simulink model "proiect_date_modificateV2"  (R2022b)
settings: Solver=VariableStepAuto  StartTime=0.0  StopTime=2500  RelTol=1e-3
values from neighbouring files (symbols this model uses):
  C = 9    [Coeficienti_Pompa.m]    (also in Coeficienti_Pompa_Modificati.m = 5.75; Coeficienti_Pompa_ModificatiV2.m = 7.55)
  k = 0.035    [Coeficienti_Pompa.m]    (also in Coeficienti_Pompa_Modificati.m = 0.025; Coeficienti_Pompa_ModificatiV2.m = 0.037)
  k1 = 0.624    [Coeficienti_Pompa.m]    (also in Coeficienti_Pompa_Modificati.m; Coeficienti_Pompa_ModificatiV2.m)
  k11 = k2^2 + 4* (k - k3) * k1    (= 0.0890826)    [Coeficienti_Pompa.m]    (also in Coeficienti_Pompa_Modificati.m = 0.0641226; Coeficienti_Pompa_ModificatiV2.m = 0.0940746)
  k12 = 8* (k - k3) * h    (= 0.2848)    [Coeficienti_Pompa.m]    (also in Coeficienti_Pompa_Modificati.m = 0.2048; Coeficienti_Pompa_ModificatiV2.m = 0.3008)
  k13 = 2* (k - k3)    (= 0.0712)    [Coeficienti_Pompa.m]    (also in Coeficienti_Pompa_Modificati.m = 0.0512; Coeficienti_Pompa_ModificatiV2.m = 0.0752)
  k2 = -0.015    [Coeficienti_Pompa.m]    (also in Coeficienti_Pompa_Modificati.m; Coeficienti_Pompa_ModificatiV2.m)
  k3 = -0.0006    [Coeficienti_Pompa.m]    (also in Coeficienti_Pompa_Modificati.m; Coeficienti_Pompa_ModificatiV2.m)
  kcompensare = (deltah/deltaq)/(deltah/deltau)    (= 0.1)    [Coeficienti_Pompa.m]    (also in Coeficienti_Pompa_Modificati.m; Coeficienti_Pompa_ModificatiV2.m)
  keta = 8e-5    (= 8e-05)    [Coeficienti_Pompa.m]    (also in Coeficienti_Pompa_Modificati.m; Coeficienti_Pompa_ModificatiV2.m)
libraries: slpidlib x7
(part 1 of 2)
settings Model: Creator=bn19b  LastModifiedBy=bn19b

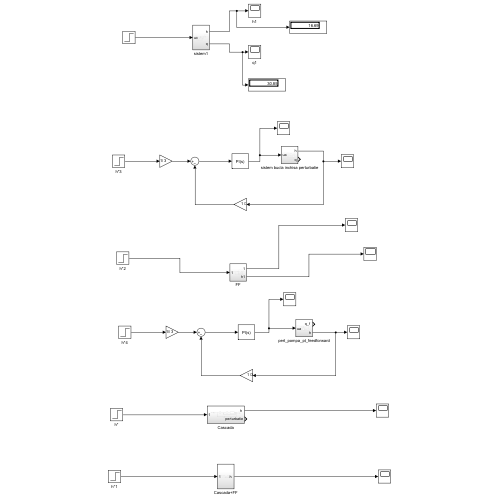
[thumbnail: Simulink's stored preview of the top-level diagram]
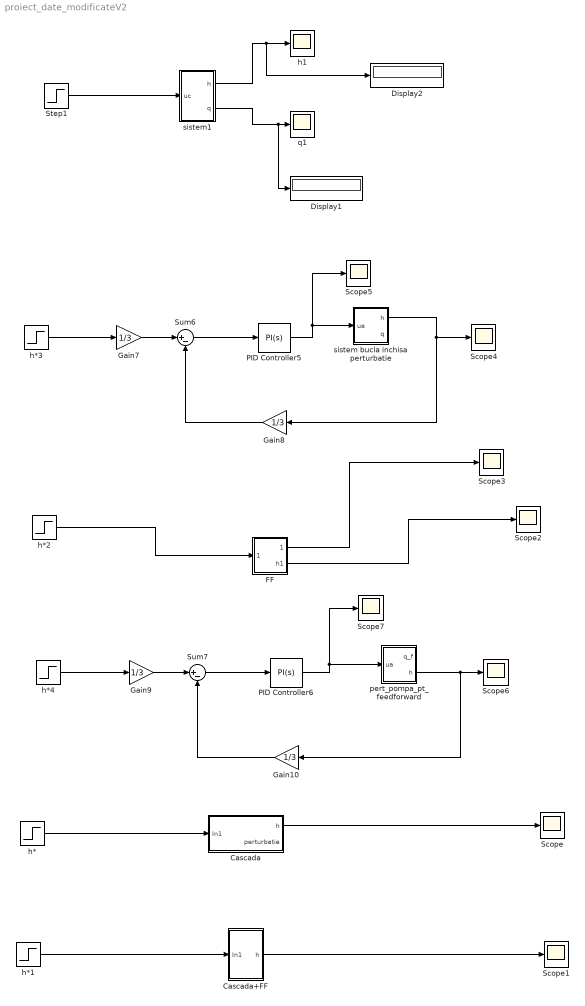
== system proiect_date_modificateV2 ==
  Cascada : Subsystem
  Cascada+FF : Subsystem
  Display1 : Display
  Display2 : Display
  FF : Subsystem
  Gain{7..10} (4 alike) : Gain  Gain=1/3
  PID Controller5 : slpidlib/PID Controller  Controller=PI  Form=Parallel  TimeDomain=Continuous-time  UseExternalTs=off  SampleTime=-1  IntegratorMethod=Forward Euler  FilterMethod=Forward Euler  ControllerParametersSource=internal  P=0.164  I=0.00129  UseKiTs=off  D=0  N=100  UseFilter=on  TunerSelectOption=Transfer Function Based (PID Tuner App)  InitialConditionSource=internal  InitialConditionForIntegrator=5  InitialConditionForFilter=0  DifferentiatorICPrevScaledInput=0  ExternalReset=none  TrackingMode=off  Kt=1  LimitOutput=off  SatLimitsSource=internal  UpperSaturationLimit=inf  LowerSaturationLimit=-inf  LinearizeAsGain=on  AntiWindupMode=none  Kb=1  LimitIntegrator=off  UpperIntegratorSaturationLimit=inf  LowerIntegratorSaturationLimit=-inf  POutMin=[]  POutMax=[]  IOutMin=[]  IOutMax=[]  DOutMin=[]  DOutMax=[]  NOutMin=[]  NOutMax=[]  SumOutMin=[]  SumOutMax=[]  SaturationOutMin=[]  SaturationOutMax=[]  PParamMin=[]  PParamMax=[]  IParamMin=[]  IParamMax=[]  DParamMin=[]  DParamMax=[]  NParamMin=[]  NParamMax=[]  KbParamMin=[]  KbParamMax=[]  KtParamMin=[]  KtParamMax=[]  KbOutMin=[]  KbOutMax=[]  KtOutMin=[]  KtOutMax=[]  IntegratorOutMin=[]  IntegratorOutMax=[]  FilterOutMin=[]  FilterOutMax=[]  SumI1OutMin=[]  SumI1OutMax=[]  SumI2OutMin=[]  SumI2OutMax=[]  SumI3OutMin=[]  SumI3OutMax=[]  SumI4OutMin=[]  SumI4OutMax=[]  SumDOutMin=[]  SumDOutMax=[]  DifferentiatorOutMin=[]  DifferentiatorOutMax=[]  FilterDiffOutCoefMin=[]  FilterDiffOutCoefMax=[]  ReciprocalOutMin=[]  ReciprocalOutMax=[]  SumDenOutMin=[]  SumDenOutMax=[]  SumNumOutMin=[]  SumNumOutMax=[]  DivideOutMin=[]  DivideOutMax=[]  UdiffTsProdOutMin=[]  UdiffTsProdOutMax=[]  NTsProdOutMin=[]  NTsProdOutMax=[]  UintegralTsProdOutMin=[]  UintegralTsProdOutMax=[]  UngainTsProdOutMin=[]  UngainTsProdOutMax=[]  ClampingZeroOutDataTypeStr=Inherit: Inherit via back propagation  ClampingZeroOutMin=[]  ClampingZeroOutMax=[]  FilterDenConstantOutDataTypeStr=Inherit: Inherit via back propagation  FilterDenConstantOutMin=[]  FilterDenConstantOutMax=[]  PCopyOutDataTypeStr=Inherit: Inherit via back propagation  PCopyOutMin=[]  PCopyOutMax=[]  NCopyOutDataTypeStr=Inherit: Inherit via back propagation  NCopyOutMin=[]  NCopyOutMax=[]  IntegratorContinuousStateAttributes=''  IntegratorStateMustResolveToSignalObject=off  IntegratorRTWStateStorageClass=Auto  FilterContinuousStateAttributes=''  FilterStateMustResolveToSignalObject=off  FilterRTWStateStorageClass=Auto  ParallelPVariant=InternalParameters  IdealPVariant=Disabled  IVariant=InternalParameters  DVariant=Disabled  IntegratorVariant=Continuous  SatVariant=Disabled  AWVariant=Passthrough  PCopyVariant=Disabled  TRVariant=Disabled  FdbkBlocksVariant=Forward  IdealPFdbkVariant=Disabled  SatFdbkVariant=Disabled  DerivativeFilterVariant=Disabled  NVariant=Disabled  NCopyVariant=Disabled_SignalSpec  FilterICVariant=Disabled  IntegratorICVariant=InternalICs  ExternalResetVariant=Disabled  TRSumVariant=Passthrough  SumFdbkVariant=Disabled  SumVariant=Sum_PI  TsampFilterVariant=InternalTs  TsampNgainVariant=Passthrough  TsampIntegralVariant=Passthrough  ExternalSaturationOutDataTypeStr=Inherit: Same as second input
  PID Controller6 : slpidlib/PID Controller  Controller=PI  Form=Parallel  TimeDomain=Continuous-time  UseExternalTs=off  SampleTime=-1  IntegratorMethod=Forward Euler  FilterMethod=Forward Euler  ControllerParametersSource=internal  P=0.164  I=0.00129  UseKiTs=off  D=0  N=100  UseFilter=on  TunerSelectOption=Transfer Function Based (PID Tuner App)  InitialConditionSource=internal  InitialConditionForIntegrator=5  InitialConditionForFilter=0  DifferentiatorICPrevScaledInput=0  ExternalReset=none  TrackingMode=off  Kt=1  LimitOutput=off  SatLimitsSource=internal  UpperSaturationLimit=inf  LowerSaturationLimit=-inf  LinearizeAsGain=on  AntiWindupMode=none  Kb=1  LimitIntegrator=off  UpperIntegratorSaturationLimit=inf  LowerIntegratorSaturationLimit=-inf  POutMin=[]  POutMax=[]  IOutMin=[]  IOutMax=[]  DOutMin=[]  DOutMax=[]  NOutMin=[]  NOutMax=[]  SumOutMin=[]  SumOutMax=[]  SaturationOutMin=[]  SaturationOutMax=[]  PParamMin=[]  PParamMax=[]  IParamMin=[]  IParamMax=[]  DParamMin=[]  DParamMax=[]  NParamMin=[]  NParamMax=[]  KbParamMin=[]  KbParamMax=[]  KtParamMin=[]  KtParamMax=[]  KbOutMin=[]  KbOutMax=[]  KtOutMin=[]  KtOutMax=[]  IntegratorOutMin=[]  IntegratorOutMax=[]  FilterOutMin=[]  FilterOutMax=[]  SumI1OutMin=[]  SumI1OutMax=[]  SumI2OutMin=[]  SumI2OutMax=[]  SumI3OutMin=[]  SumI3OutMax=[]  SumI4OutMin=[]  SumI4OutMax=[]  SumDOutMin=[]  SumDOutMax=[]  DifferentiatorOutMin=[]  DifferentiatorOutMax=[]  FilterDiffOutCoefMin=[]  FilterDiffOutCoefMax=[]  ReciprocalOutMin=[]  ReciprocalOutMax=[]  SumDenOutMin=[]  SumDenOutMax=[]  SumNumOutMin=[]  SumNumOutMax=[]  DivideOutMin=[]  DivideOutMax=[]  UdiffTsProdOutMin=[]  UdiffTsProdOutMax=[]  NTsProdOutMin=[]  NTsProdOutMax=[]  UintegralTsProdOutMin=[]  UintegralTsProdOutMax=[]  UngainTsProdOutMin=[]  UngainTsProdOutMax=[]  ClampingZeroOutDataTypeStr=Inherit: Inherit via back propagation  ClampingZeroOutMin=[]  ClampingZeroOutMax=[]  FilterDenConstantOutDataTypeStr=Inherit: Inherit via back propagation  FilterDenConstantOutMin=[]  FilterDenConstantOutMax=[]  PCopyOutDataTypeStr=Inherit: Inherit via back propagation  PCopyOutMin=[]  PCopyOutMax=[]  NCopyOutDataTypeStr=Inherit: Inherit via back propagation  NCopyOutMin=[]  NCopyOutMax=[]  IntegratorContinuousStateAttributes=''  IntegratorStateMustResolveToSignalObject=off  IntegratorRTWStateStorageClass=Auto  FilterContinuousStateAttributes=''  FilterStateMustResolveToSignalObject=off  FilterRTWStateStorageClass=Auto  ParallelPVariant=InternalParameters  IdealPVariant=Disabled  IVariant=InternalParameters  DVariant=Disabled  IntegratorVariant=Continuous  SatVariant=Disabled  AWVariant=Passthrough  PCopyVariant=Disabled  TRVariant=Disabled  FdbkBlocksVariant=Forward  IdealPFdbkVariant=Disabled  SatFdbkVariant=Disabled  DerivativeFilterVariant=Disabled  NVariant=Disabled  NCopyVariant=Disabled_SignalSpec  FilterICVariant=Disabled  IntegratorICVariant=InternalICs  ExternalResetVariant=Disabled  TRSumVariant=Passthrough  SumFdbkVariant=Disabled  SumVariant=Sum_PI  TsampFilterVariant=InternalTs  TsampNgainVariant=Passthrough  TsampIntegralVariant=Passthrough  ExternalSaturationOutDataTypeStr=Inherit: Same as second input
  Scope{,1..7} (8 alike) : Scope
  Step1 : Step  After=5.7  SampleTime=0
  Sum6 : Sum  Inputs=|+-
  Sum7 : Sum  Inputs=|+-
  h*{,1..4} (5 alike) : Step  Before=16.69  After=20.85  SampleTime=0
  h1 : Scope
  pert_pompa_pt_feedforward : Subsystem
  q1 : Scope
  sistem bucla inchisa perturbatie : Subsystem
  sistem1 : Subsystem
  wires:
  Sum6/1 -> PID Controller5/1
  sistem bucla inchisa perturbatie/1(h) -> Gain8/1, Scope4/1
  pert_pompa_pt_feedforward/2(h) -> Gain10/1, Scope6/1
  Gain10/1 -> Sum7/2
  sistem1/2(q) -> Display1/1, q1/1
  PID Controller6/1 -> pert_pompa_pt_feedforward/1(ua), Scope7/1
  h*2/1 -> FF/1(In1)
  PID Controller5/1 -> sistem bucla inchisa perturbatie/1(ua), Scope5/1
  h*3/1 -> Gain7/1
  Sum7/1 -> PID Controller6/1
  Gain7/1 -> Sum6/1
  FF/2(h1) -> Scope2/1
  sistem1/1(h) -> Display2/1, h1/1
  h*4/1 -> Gain9/1
  Gain9/1 -> Sum7/1
  FF/1(Out1) -> Scope3/1
  Step1/1 -> sistem1/1(uc)
  Gain8/1 -> Sum6/2
  h*/1 -> Cascada/1(In1)
  Cascada/1("h ") -> Scope/1
  Cascada+FF/1("h ") -> Scope1/1
  h*1/1 -> Cascada+FF/1(In1)

== system proiect_date_modificateV2/Cascada ==
  In1 : Inport
  Gain : Gain  Gain=1/3
  Gain1 : Gain  Gain=1/3
  PID Controller : slpidlib/PID Controller  Controller=PI  Form=Parallel  TimeDomain=Continuous-time  UseExternalTs=off  SampleTime=-1  IntegratorMethod=Forward Euler  FilterMethod=Forward Euler  ControllerParametersSource=internal  P=0.0189  I=8.46e-05  UseKiTs=off  D=0  N=100  UseFilter=on  TunerSelectOption=Transfer Function Based (PID Tuner App)  InitialConditionSource=internal  InitialConditionForIntegrator=29.2  InitialConditionForFilter=0  DifferentiatorICPrevScaledInput=0  ExternalReset=none  TrackingMode=off  Kt=1  LimitOutput=off  SatLimitsSource=internal  UpperSaturationLimit=inf  LowerSaturationLimit=-inf  LinearizeAsGain=on  AntiWindupMode=none  Kb=1  LimitIntegrator=off  UpperIntegratorSaturationLimit=inf  LowerIntegratorSaturationLimit=-inf  POutMin=[]  POutMax=[]  IOutMin=[]  IOutMax=[]  DOutMin=[]  DOutMax=[]  NOutMin=[]  NOutMax=[]  SumOutMin=[]  SumOutMax=[]  SaturationOutMin=[]  SaturationOutMax=[]  PParamMin=[]  PParamMax=[]  IParamMin=[]  IParamMax=[]  DParamMin=[]  DParamMax=[]  NParamMin=[]  NParamMax=[]  KbParamMin=[]  KbParamMax=[]  KtParamMin=[]  KtParamMax=[]  KbOutMin=[]  KbOutMax=[]  KtOutMin=[]  KtOutMax=[]  IntegratorOutMin=[]  IntegratorOutMax=[]  FilterOutMin=[]  FilterOutMax=[]  SumI1OutMin=[]  SumI1OutMax=[]  SumI2OutMin=[]  SumI2OutMax=[]  SumI3OutMin=[]  SumI3OutMax=[]  SumI4OutMin=[]  SumI4OutMax=[]  SumDOutMin=[]  SumDOutMax=[]  DifferentiatorOutMin=[]  DifferentiatorOutMax=[]  FilterDiffOutCoefMin=[]  FilterDiffOutCoefMax=[]  ReciprocalOutMin=[]  ReciprocalOutMax=[]  SumDenOutMin=[]  SumDenOutMax=[]  SumNumOutMin=[]  SumNumOutMax=[]  DivideOutMin=[]  DivideOutMax=[]  UdiffTsProdOutMin=[]  UdiffTsProdOutMax=[]  NTsProdOutMin=[]  NTsProdOutMax=[]  UintegralTsProdOutMin=[]  UintegralTsProdOutMax=[]  UngainTsProdOutMin=[]  UngainTsProdOutMax=[]  ClampingZeroOutDataTypeStr=Inherit: Inherit via back propagation  ClampingZeroOutMin=[]  ClampingZeroOutMax=[]  FilterDenConstantOutDataTypeStr=Inherit: Inherit via back propagation  FilterDenConstantOutMin=[]  FilterDenConstantOutMax=[]  PCopyOutDataTypeStr=Inherit: Inherit via back propagation  PCopyOutMin=[]  PCopyOutMax=[]  NCopyOutDataTypeStr=Inherit: Inherit via back propagation  NCopyOutMin=[]  NCopyOutMax=[]  IntegratorContinuousStateAttributes=''  IntegratorStateMustResolveToSignalObject=off  IntegratorRTWStateStorageClass=Auto  FilterContinuousStateAttributes=''  FilterStateMustResolveToSignalObject=off  FilterRTWStateStorageClass=Auto  ParallelPVariant=InternalParameters  IdealPVariant=Disabled  IVariant=InternalParameters  DVariant=Disabled  IntegratorVariant=Continuous  SatVariant=Disabled  AWVariant=Passthrough  PCopyVariant=Disabled  TRVariant=Disabled  FdbkBlocksVariant=Forward  IdealPFdbkVariant=Disabled  SatFdbkVariant=Disabled  DerivativeFilterVariant=Disabled  NVariant=Disabled  NCopyVariant=Disabled_SignalSpec  FilterICVariant=Disabled  IntegratorICVariant=InternalICs  ExternalResetVariant=Disabled  TRSumVariant=Passthrough  SumFdbkVariant=Disabled  SumVariant=Sum_PI  TsampFilterVariant=InternalTs  TsampNgainVariant=Passthrough  TsampIntegralVariant=Passthrough  ExternalSaturationOutDataTypeStr=Inherit: Same as second input
  PID Controller2 : slpidlib/PID Controller  Controller=PI  Form=Parallel  TimeDomain=Continuous-time  UseExternalTs=off  SampleTime=-1  IntegratorMethod=Forward Euler  FilterMethod=Forward Euler  ControllerParametersSource=internal  P=4.74  I=6.49  UseKiTs=off  D=0  N=100  UseFilter=on  TunerSelectOption=Transfer Function Based (PID Tuner App)  InitialConditionSource=internal  InitialConditionForIntegrator=uc  InitialConditionForFilter=0  DifferentiatorICPrevScaledInput=0  ExternalReset=none  TrackingMode=off  Kt=1  LimitOutput=off  SatLimitsSource=internal  UpperSaturationLimit=inf  LowerSaturationLimit=-inf  LinearizeAsGain=on  AntiWindupMode=none  Kb=1  LimitIntegrator=off  UpperIntegratorSaturationLimit=inf  LowerIntegratorSaturationLimit=-inf  POutMin=[]  POutMax=[]  IOutMin=[]  IOutMax=[]  DOutMin=[]  DOutMax=[]  NOutMin=[]  NOutMax=[]  SumOutMin=[]  SumOutMax=[]  SaturationOutMin=[]  SaturationOutMax=[]  PParamMin=[]  PParamMax=[]  IParamMin=[]  IParamMax=[]  DParamMin=[]  DParamMax=[]  NParamMin=[]  NParamMax=[]  KbParamMin=[]  KbParamMax=[]  KtParamMin=[]  KtParamMax=[]  KbOutMin=[]  KbOutMax=[]  KtOutMin=[]  KtOutMax=[]  IntegratorOutMin=[]  IntegratorOutMax=[]  FilterOutMin=[]  FilterOutMax=[]  SumI1OutMin=[]  SumI1OutMax=[]  SumI2OutMin=[]  SumI2OutMax=[]  SumI3OutMin=[]  SumI3OutMax=[]  SumI4OutMin=[]  SumI4OutMax=[]  SumDOutMin=[]  SumDOutMax=[]  DifferentiatorOutMin=[]  DifferentiatorOutMax=[]  FilterDiffOutCoefMin=[]  FilterDiffOutCoefMax=[]  ReciprocalOutMin=[]  ReciprocalOutMax=[]  SumDenOutMin=[]  SumDenOutMax=[]  SumNumOutMin=[]  SumNumOutMax=[]  DivideOutMin=[]  DivideOutMax=[]  UdiffTsProdOutMin=[]  UdiffTsProdOutMax=[]  NTsProdOutMin=[]  NTsProdOutMax=[]  UintegralTsProdOutMin=[]  UintegralTsProdOutMax=[]  UngainTsProdOutMin=[]  UngainTsProdOutMax=[]  ClampingZeroOutDataTypeStr=Inherit: Inherit via back propagation  ClampingZeroOutMin=[]  ClampingZeroOutMax=[]  FilterDenConstantOutDataTypeStr=Inherit: Inherit via back propagation  FilterDenConstantOutMin=[]  FilterDenConstantOutMax=[]  PCopyOutDataTypeStr=Inherit: Inherit via back propagation  PCopyOutMin=[]  PCopyOutMax=[]  NCopyOutDataTypeStr=Inherit: Inherit via back propagation  NCopyOutMin=[]  NCopyOutMax=[]  IntegratorContinuousStateAttributes=''  IntegratorStateMustResolveToSignalObject=off  IntegratorRTWStateStorageClass=Auto  FilterContinuousStateAttributes=''  FilterStateMustResolveToSignalObject=off  FilterRTWStateStorageClass=Auto  ParallelPVariant=InternalParameters  IdealPVariant=Disabled  IVariant=InternalParameters  DVariant=Disabled  IntegratorVariant=Continuous  SatVariant=Disabled  AWVariant=Passthrough  PCopyVariant=Disabled  TRVariant=Disabled  FdbkBlocksVariant=Forward  IdealPFdbkVariant=Disabled  SatFdbkVariant=Disabled  DerivativeFilterVariant=Disabled  NVariant=Disabled  NCopyVariant=Disabled_SignalSpec  FilterICVariant=Disabled  IntegratorICVariant=InternalICs  ExternalResetVariant=Disabled  TRSumVariant=Passthrough  SumFdbkVariant=Disabled  SumVariant=Sum_PI  TsampFilterVariant=InternalTs  TsampNgainVariant=Passthrough  TsampIntegralVariant=Passthrough  ExternalSaturationOutDataTypeStr=Inherit: Same as second input
  Sum : Sum  Inputs=|+-
  Sum1 : Sum  Inputs=|+-
  sistem_cascada : Subsystem
  "h " : Outport
  perturbatie : Outport  Port=2
  wires:
  Gain/1 -> Sum/1
  PID Controller/1 -> Sum1/1
  Sum1/1 -> PID Controller2/1
  sistem_cascada/3(q1) -> Sum1/2
  Sum/1 -> PID Controller/1
  sistem_cascada/1("h ") -> "h "/1, Gain1/1
  PID Controller2/1 -> sistem_cascada/1(uc)
  Gain1/1 -> Sum/2
  In1/1 -> Gain/1
  sistem_cascada/2(perturbatie) -> perturbatie/1

== system proiect_date_modificateV2/Cascada+FF ==
  In1 : Inport
  Gain2 : Gain  Gain=1/3
  Gain3 : Gain  Gain=1/3
  PID Controller1 : slpidlib/PID Controller  Controller=PI  Form=Parallel  TimeDomain=Continuous-time  UseExternalTs=off  SampleTime=-1  IntegratorMethod=Forward Euler  FilterMethod=Forward Euler  ControllerParametersSource=internal  P=0.0189  I=8.46e-05  UseKiTs=off  D=0  N=100  UseFilter=on  TunerSelectOption=Transfer Function Based (PID Tuner App)  InitialConditionSource=internal  InitialConditionForIntegrator=29.2  InitialConditionForFilter=0  DifferentiatorICPrevScaledInput=0  ExternalReset=none  TrackingMode=off  Kt=1  LimitOutput=off  SatLimitsSource=internal  UpperSaturationLimit=inf  LowerSaturationLimit=-inf  LinearizeAsGain=on  AntiWindupMode=none  Kb=1  LimitIntegrator=off  UpperIntegratorSaturationLimit=inf  LowerIntegratorSaturationLimit=-inf  POutMin=[]  POutMax=[]  IOutMin=[]  IOutMax=[]  DOutMin=[]  DOutMax=[]  NOutMin=[]  NOutMax=[]  SumOutMin=[]  SumOutMax=[]  SaturationOutMin=[]  SaturationOutMax=[]  PParamMin=[]  PParamMax=[]  IParamMin=[]  IParamMax=[]  DParamMin=[]  DParamMax=[]  NParamMin=[]  NParamMax=[]  KbParamMin=[]  KbParamMax=[]  KtParamMin=[]  KtParamMax=[]  KbOutMin=[]  KbOutMax=[]  KtOutMin=[]  KtOutMax=[]  IntegratorOutMin=[]  IntegratorOutMax=[]  FilterOutMin=[]  FilterOutMax=[]  SumI1OutMin=[]  SumI1OutMax=[]  SumI2OutMin=[]  SumI2OutMax=[]  SumI3OutMin=[]  SumI3OutMax=[]  SumI4OutMin=[]  SumI4OutMax=[]  SumDOutMin=[]  SumDOutMax=[]  DifferentiatorOutMin=[]  DifferentiatorOutMax=[]  FilterDiffOutCoefMin=[]  FilterDiffOutCoefMax=[]  ReciprocalOutMin=[]  ReciprocalOutMax=[]  SumDenOutMin=[]  SumDenOutMax=[]  SumNumOutMin=[]  SumNumOutMax=[]  DivideOutMin=[]  DivideOutMax=[]  UdiffTsProdOutMin=[]  UdiffTsProdOutMax=[]  NTsProdOutMin=[]  NTsProdOutMax=[]  UintegralTsProdOutMin=[]  UintegralTsProdOutMax=[]  UngainTsProdOutMin=[]  UngainTsProdOutMax=[]  ClampingZeroOutDataTypeStr=Inherit: Inherit via back propagation  ClampingZeroOutMin=[]  ClampingZeroOutMax=[]  FilterDenConstantOutDataTypeStr=Inherit: Inherit via back propagation  FilterDenConstantOutMin=[]  FilterDenConstantOutMax=[]  PCopyOutDataTypeStr=Inherit: Inherit via back propagation  PCopyOutMin=[]  PCopyOutMax=[]  NCopyOutDataTypeStr=Inherit: Inherit via back propagation  NCopyOutMin=[]  NCopyOutMax=[]  IntegratorContinuousStateAttributes=''  IntegratorStateMustResolveToSignalObject=off  IntegratorRTWStateStorageClass=Auto  FilterContinuousStateAttributes=''  FilterStateMustResolveToSignalObject=off  FilterRTWStateStorageClass=Auto  ParallelPVariant=InternalParameters  IdealPVariant=Disabled  IVariant=InternalParameters  DVariant=Disabled  IntegratorVariant=Continuous  SatVariant=Disabled  AWVariant=Passthrough  PCopyVariant=Disabled  TRVariant=Disabled  FdbkBlocksVariant=Forward  IdealPFdbkVariant=Disabled  SatFdbkVariant=Disabled  DerivativeFilterVariant=Disabled  NVariant=Disabled  NCopyVariant=Disabled_SignalSpec  FilterICVariant=Disabled  IntegratorICVariant=InternalICs  ExternalResetVariant=Disabled  TRSumVariant=Passthrough  SumFdbkVariant=Disabled  SumVariant=Sum_PI  TsampFilterVariant=InternalTs  TsampNgainVariant=Passthrough  TsampIntegralVariant=Passthrough  ExternalSaturationOutDataTypeStr=Inherit: Same as second input
  PID Controller3 : slpidlib/PID Controller  Controller=PI  Form=Parallel  TimeDomain=Continuous-time  UseExternalTs=off  SampleTime=-1  IntegratorMethod=Forward Euler  FilterMethod=Forward Euler  ControllerParametersSource=internal  P=4.74  I=6.49  UseKiTs=off  D=0  N=100  UseFilter=on  TunerSelectOption=Transfer Function Based (PID Tuner App)  InitialConditionSource=internal  InitialConditionForIntegrator=5  InitialConditionForFilter=0  DifferentiatorICPrevScaledInput=0  ExternalReset=none  TrackingMode=off  Kt=1  LimitOutput=off  SatLimitsSource=internal  UpperSaturationLimit=inf  LowerSaturationLimit=-inf  LinearizeAsGain=on  AntiWindupMode=none  Kb=1  LimitIntegrator=off  UpperIntegratorSaturationLimit=inf  LowerIntegratorSaturationLimit=-inf  POutMin=[]  POutMax=[]  IOutMin=[]  IOutMax=[]  DOutMin=[]  DOutMax=[]  NOutMin=[]  NOutMax=[]  SumOutMin=[]  SumOutMax=[]  SaturationOutMin=[]  SaturationOutMax=[]  PParamMin=[]  PParamMax=[]  IParamMin=[]  IParamMax=[]  DParamMin=[]  DParamMax=[]  NParamMin=[]  NParamMax=[]  KbParamMin=[]  KbParamMax=[]  KtParamMin=[]  KtParamMax=[]  KbOutMin=[]  KbOutMax=[]  KtOutMin=[]  KtOutMax=[]  IntegratorOutMin=[]  IntegratorOutMax=[]  FilterOutMin=[]  FilterOutMax=[]  SumI1OutMin=[]  SumI1OutMax=[]  SumI2OutMin=[]  SumI2OutMax=[]  SumI3OutMin=[]  SumI3OutMax=[]  SumI4OutMin=[]  SumI4OutMax=[]  SumDOutMin=[]  SumDOutMax=[]  DifferentiatorOutMin=[]  DifferentiatorOutMax=[]  FilterDiffOutCoefMin=[]  FilterDiffOutCoefMax=[]  ReciprocalOutMin=[]  ReciprocalOutMax=[]  SumDenOutMin=[]  SumDenOutMax=[]  SumNumOutMin=[]  SumNumOutMax=[]  DivideOutMin=[]  DivideOutMax=[]  UdiffTsProdOutMin=[]  UdiffTsProdOutMax=[]  NTsProdOutMin=[]  NTsProdOutMax=[]  UintegralTsProdOutMin=[]  UintegralTsProdOutMax=[]  UngainTsProdOutMin=[]  UngainTsProdOutMax=[]  ClampingZeroOutDataTypeStr=Inherit: Inherit via back propagation  ClampingZeroOutMin=[]  ClampingZeroOutMax=[]  FilterDenConstantOutDataTypeStr=Inherit: Inherit via back propagation  FilterDenConstantOutMin=[]  FilterDenConstantOutMax=[]  PCopyOutDataTypeStr=Inherit: Inherit via back propagation  PCopyOutMin=[]  PCopyOutMax=[]  NCopyOutDataTypeStr=Inherit: Inherit via back propagation  NCopyOutMin=[]  NCopyOutMax=[]  IntegratorContinuousStateAttributes=''  IntegratorStateMustResolveToSignalObject=off  IntegratorRTWStateStorageClass=Auto  FilterContinuousStateAttributes=''  FilterStateMustResolveToSignalObject=off  FilterRTWStateStorageClass=Auto  ParallelPVariant=InternalParameters  IdealPVariant=Disabled  IVariant=InternalParameters  DVariant=Disabled  IntegratorVariant=Continuous  SatVariant=Disabled  AWVariant=Passthrough  PCopyVariant=Disabled  TRVariant=Disabled  FdbkBlocksVariant=Forward  IdealPFdbkVariant=Disabled  SatFdbkVariant=Disabled  DerivativeFilterVariant=Disabled  NVariant=Disabled  NCopyVariant=Disabled_SignalSpec  FilterICVariant=Disabled  IntegratorICVariant=InternalICs  ExternalResetVariant=Disabled  TRSumVariant=Passthrough  SumFdbkVariant=Disabled  SumVariant=Sum_PI  TsampFilterVariant=InternalTs  TsampNgainVariant=Passthrough  TsampIntegralVariant=Passthrough  ExternalSaturationOutDataTypeStr=Inherit: Same as second input
  Sum2 : Sum  Inputs=|+-
  Sum3 : Sum  Inputs=|++-
  cascada+ff : Subsystem
  "h " : Outport
  wires:
  cascada+ff/2(perturbatie) -> Sum3/2
  Gain3/1 -> Sum2/2
  cascada+ff/1("h ") -> "h "/1, Gain3/1
  Sum3/1 -> PID Controller3/1
  Gain2/1 -> Sum2/1
  cascada+ff/3(q1) -> Sum3/3
  PID Controller3/1 -> cascada+ff/1(uc)
  PID Controller1/1 -> Sum3/1
  Sum2/1 -> PID Controller1/1
  In1/1 -> Gain2/1

== system proiect_date_modificateV2/FF ==
  In1 : Inport
  Gain4 : Gain  Gain=1/3
  Gain5 : Gain  Gain=1/3
  Gain6 : Gain  Gain=kcompensare
  PID Controller4 : slpidlib/PID Controller  Controller=PI  Form=Parallel  TimeDomain=Continuous-time  UseExternalTs=off  SampleTime=-1  IntegratorMethod=Forward Euler  FilterMethod=Forward Euler  ControllerParametersSource=internal  P=0.164  I=0.00129  UseKiTs=off  D=0  N=100  UseFilter=on  TunerSelectOption=Transfer Function Based (PID Tuner App)  InitialConditionSource=internal  InitialConditionForIntegrator=5  InitialConditionForFilter=0  DifferentiatorICPrevScaledInput=0  ExternalReset=none  TrackingMode=off  Kt=1  LimitOutput=off  SatLimitsSource=internal  UpperSaturationLimit=inf  LowerSaturationLimit=-inf  LinearizeAsGain=on  AntiWindupMode=none  Kb=1  LimitIntegrator=off  UpperIntegratorSaturationLimit=inf  LowerIntegratorSaturationLimit=-inf  POutMin=[]  POutMax=[]  IOutMin=[]  IOutMax=[]  DOutMin=[]  DOutMax=[]  NOutMin=[]  NOutMax=[]  SumOutMin=[]  SumOutMax=[]  SaturationOutMin=[]  SaturationOutMax=[]  PParamMin=[]  PParamMax=[]  IParamMin=[]  IParamMax=[]  DParamMin=[]  DParamMax=[]  NParamMin=[]  NParamMax=[]  KbParamMin=[]  KbParamMax=[]  KtParamMin=[]  KtParamMax=[]  KbOutMin=[]  KbOutMax=[]  KtOutMin=[]  KtOutMax=[]  IntegratorOutMin=[]  IntegratorOutMax=[]  FilterOutMin=[]  FilterOutMax=[]  SumI1OutMin=[]  SumI1OutMax=[]  SumI2OutMin=[]  SumI2OutMax=[]  SumI3OutMin=[]  SumI3OutMax=[]  SumI4OutMin=[]  SumI4OutMax=[]  SumDOutMin=[]  SumDOutMax=[]  DifferentiatorOutMin=[]  DifferentiatorOutMax=[]  FilterDiffOutCoefMin=[]  FilterDiffOutCoefMax=[]  ReciprocalOutMin=[]  ReciprocalOutMax=[]  SumDenOutMin=[]  SumDenOutMax=[]  SumNumOutMin=[]  SumNumOutMax=[]  DivideOutMin=[]  DivideOutMax=[]  UdiffTsProdOutMin=[]  UdiffTsProdOutMax=[]  NTsProdOutMin=[]  NTsProdOutMax=[]  UintegralTsProdOutMin=[]  UintegralTsProdOutMax=[]  UngainTsProdOutMin=[]  UngainTsProdOutMax=[]  ClampingZeroOutDataTypeStr=Inherit: Inherit via back propagation  ClampingZeroOutMin=[]  ClampingZeroOutMax=[]  FilterDenConstantOutDataTypeStr=Inherit: Inherit via back propagation  FilterDenConstantOutMin=[]  FilterDenConstantOutMax=[]  PCopyOutDataTypeStr=Inherit: Inherit via back propagation  PCopyOutMin=[]  PCopyOutMax=[]  NCopyOutDataTypeStr=Inherit: Inherit via back propagation  NCopyOutMin=[]  NCopyOutMax=[]  IntegratorContinuousStateAttributes=''  IntegratorStateMustResolveToSignalObject=off  IntegratorRTWStateStorageClass=Auto  FilterContinuousStateAttributes=''  FilterStateMustResolveToSignalObject=off  FilterRTWStateStorageClass=Auto  ParallelPVariant=InternalParameters  IdealPVariant=Disabled  IVariant=InternalParameters  DVariant=Disabled  IntegratorVariant=Continuous  SatVariant=Disabled  AWVariant=Passthrough  PCopyVariant=Disabled  TRVariant=Disabled  FdbkBlocksVariant=Forward  IdealPFdbkVariant=Disabled  SatFdbkVariant=Disabled  DerivativeFilterVariant=Disabled  NVariant=Disabled  NCopyVariant=Disabled_SignalSpec  FilterICVariant=Disabled  IntegratorICVariant=InternalICs  ExternalResetVariant=Disabled  TRSumVariant=Passthrough  SumFdbkVariant=Disabled  SumVariant=Sum_PI  TsampFilterVariant=InternalTs  TsampNgainVariant=Passthrough  TsampIntegralVariant=Passthrough  ExternalSaturationOutDataTypeStr=Inherit: Same as second input
  Sum4 : Sum  Inputs=|+-
  Sum5 : Sum  Inputs=|++
  sistem_feedforward : Subsystem
  Out1 : Outport
  h1 : Outport  Port=2
  wires:
  sistem_feedforward/1(h1) -> h1/1, Gain5/1
  Sum4/1 -> PID Controller4/1
  Gain6/1 -> Sum5/2
  sistem_feedforward/2(perturabtie) -> Gain6/1
  Gain5/1 -> Sum4/2
  Sum5/1 -> Out1/1, sistem_feedforward/1(ua)
  PID Controller4/1 -> Sum5/1
  Gain4/1 -> Sum4/1
  In1/1 -> Gain4/1

== system proiect_date_modificateV2/pert_pompa_pt_feedforward ==
  ua : Inport
  Amplificator : Subsystem
  Curent : Subsystem
  "Filtru " : Subsystem
  Motor : Subsystem
  Randament : Subsystem
  Rezervor : Subsystem
  Step : Step  Time=250  After=0.04  SampleTime=0
  pompa_perturbatie1 : Subsystem
  "q_f " : Outport
  h : Outport  Port=2
  wires:
  Motor/1(kn) -> pompa_perturbatie1/1(kn1)
  pompa_perturbatie1/1(q1) -> "Filtru "/1(q)
  Step/1 -> pompa_perturbatie1/3(perturbatie k)
  Rezervor/1(h) -> h/1, pompa_perturbatie1/2(h1), Curent/1(h)
  "Filtru "/1("q_f ") -> "q_f "/1, Rezervor/1("q "), Randament/1(q), Curent/2(q)
  Curent/1(im) -> Motor/2(im)
  Amplificator/1(um) -> Curent/4(um), Randament/2(um), Motor/1(um)
  Randament/1(eta) -> Curent/3(eta)
  ua/1 -> Amplificator/1(ua)

== system proiect_date_modificateV2/sistem bucla inchisa perturbatie ==
  ua : Inport
  Amplificator : Subsystem
  Curent : Subsystem
  "Filtru " : Subsystem
  Motor : Subsystem
  "Pompa " : Subsystem
  Randament : Subsystem
  Rezervor cu perturbatie : Subsystem
  h : Outport
  q : Outport  Port=2
  wires:
  "Pompa "/1(q) -> "Filtru "/1(q)
  ua/1 -> Amplificator/1(ua)
  Rezervor cu perturbatie/1(h1) -> h/1, "Pompa "/2(h), Curent/1(h)
  Motor/1(kn) -> "Pompa "/1(kn)
  "Filtru "/1("q_f ") -> q/1, Rezervor cu perturbatie/1(q1), Randament/1(q), Curent/2(q)
  Amplificator/1(um) -> Curent/4(um), Randament/2(um), Motor/1(um)
  Curent/1(im) -> Motor/2(im)
  Randament/1(eta) -> Curent/3(eta)

== system proiect_date_modificateV2/sistem1 ==
  uc : Inport
  Amplificator : Subsystem
  Bazin : Subsystem
  Curent rotoric : Subsystem
  Filtru : Subsystem
  Motor : Subsystem
  Pompa : Subsystem
  Randament pompa : Subsystem
  h : Outport
  q : Outport  Port=2
  wires:
  uc/1 -> Amplificator/1(ua)
  Amplificator/1(um) -> Curent rotoric/4(um), Randament pompa/2(um), Motor/1(um)
  Curent rotoric/1(im) -> Motor/2(im)
  Motor/1(kn) -> Pompa/1(kn)
  Bazin/1(h) -> Curent rotoric/1(h), Pompa/2(h), h/1
  Filtru/1(qf) -> Curent rotoric/2(q), Randament pompa/1(q), q/1, Bazin/1(q)
  Randament pompa/1(eta) -> Curent rotoric/3(eta)
  Pompa/1(q) -> Filtru/1(q)

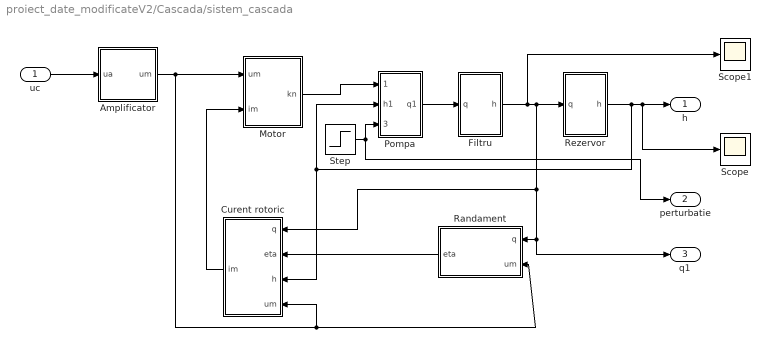
== system proiect_date_modificateV2/Cascada/sistem_cascada ==
  uc : Inport
  "Amplificator " : Subsystem
  Curent rotoric : Subsystem
  Filtru : Subsystem
  Motor : Subsystem
  Pompa : Subsystem
  Randament : Subsystem
  Rezervor : Subsystem
  Scope : Scope
  Scope1 : Scope
  Step : Step  Time=300  After=-.035  SampleTime=0
  "h " : Outport
  perturbatie : Outport  Port=2
  q1 : Outport  Port=3
  wires:
  Filtru/1(h) -> Scope1/1, Curent rotoric/1(q), q1/1, Randament/1(q), Rezervor/1(q)
  uc/1 -> "Amplificator "/1(ua)
  Randament/1(eta) -> Curent rotoric/2(eta)
  Rezervor/1(h) -> Curent rotoric/3(h), Pompa/2(h1), Scope/1, "h "/1
  Pompa/1(q1) -> Filtru/1(q)
  Curent rotoric/1(im) -> Motor/2(im)
  "Amplificator "/1(um) -> Curent rotoric/4(um), Randament/2(um), Motor/1(um)
  Motor/1(kn) -> Pompa/1(kn1)
  Step/1 -> perturbatie/1, Pompa/3(perturbatie k)

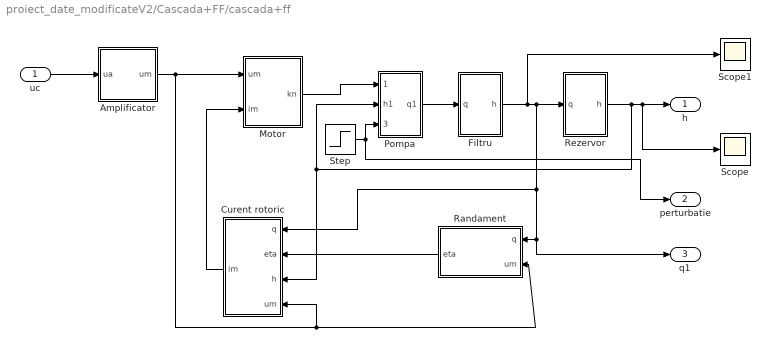
== system proiect_date_modificateV2/Cascada+FF/cascada+ff ==
  uc : Inport
  "Amplificator " : Subsystem
  Curent rotoric : Subsystem
  Filtru : Subsystem
  Motor : Subsystem
  Pompa : Subsystem
  Randament : Subsystem
  Rezervor : Subsystem
  Scope : Scope
  Scope1 : Scope
  Step : Step  Time=300  After=-.035  SampleTime=0
  "h " : Outport
  perturbatie : Outport  Port=2
  q1 : Outport  Port=3
  wires:
  Filtru/1(h) -> Scope1/1, Curent rotoric/1(q), q1/1, Randament/1(q), Rezervor/1(q)
  uc/1 -> "Amplificator "/1(ua)
  Randament/1(eta) -> Curent rotoric/2(eta)
  Rezervor/1(h) -> Curent rotoric/3(h), Pompa/2(h1), Scope/1, "h "/1
  Pompa/1(q1) -> Filtru/1(q)
  Curent rotoric/1(im) -> Motor/2(im)
  "Amplificator "/1(um) -> Curent rotoric/4(um), Randament/2(um), Motor/1(um)
  Motor/1(kn) -> Pompa/1(kn1)
  Step/1 -> perturbatie/1, Pompa/3(perturbatie k)

== system proiect_date_modificateV2/FF/sistem_feedforward ==
  ua : Inport
  Amplificator : Subsystem
  Curent : Subsystem
  "Filtru " : Subsystem
  Motor : Subsystem
  "Pompa " : Subsystem
  Randament : Subsystem
  rezervor_feedforward : Subsystem
  h1 : Outport
  perturabtie : Outport  Port=2
  wires:
  rezervor_feedforward/2(perturabtie) -> perturabtie/1
  Randament/1(eta) -> Curent/3(eta)
  Amplificator/1(um) -> Curent/4(um), Randament/2(um), Motor/1(um)
  rezervor_feedforward/1(h1) -> h1/1, "Pompa "/2(h), Curent/1(h)
  "Filtru "/1("q_f ") -> rezervor_feedforward/1(q1), Randament/1(q), Curent/2(q)
  Curent/1(im) -> Motor/2(im)
  "Pompa "/1(q) -> "Filtru "/1(q)
  ua/1 -> Amplificator/1(ua)
  Motor/1(kn) -> "Pompa "/1(kn)

== system proiect_date_modificateV2/pert_pompa_pt_feedforward/Amplificator ==
  ua : Inport
  Constant : Constant  Value=8.1
  Gain : Gain  Gain=2.2
  Gain1 : Gain  Gain=5
  Gain2 : Gain  Gain=2.2
  Saturation : Saturate  UpperLimit=22  LowerLimit=0
  Sum : Sum  Inputs=|++
  Sum1 : Sum  Inputs=|+-
  Switch : Switch  Threshold=8.1  SaturateOnIntegerOverflow=off  InputSameDT=off
  um : Outport
  wires:
  Switch/1 -> Saturation/1
  ua/1 -> Switch/2, Gain/1, Gain2/1, Sum1/1
  Sum/1 -> Switch/1
  Gain2/1 -> Sum/1
  Gain/1 -> Switch/3
  Saturation/1 -> um/1
  Gain1/1 -> Sum/2
  Sum1/1 -> Gain1/1
  Constant/1 -> Sum1/2

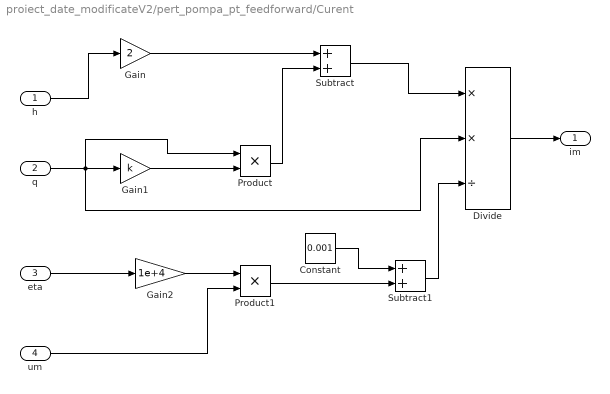
== system proiect_date_modificateV2/pert_pompa_pt_feedforward/Curent ==
  h : Inport
  q : Inport  Port=2
  eta : Inport  Port=3
  um : Inport  Port=4
  Constant : Constant  Value=0.001
  Divide : Product  Inputs=**/
  Gain : Gain  Gain=2
  Gain1 : Gain  Gain=k
  Gain2 : Gain  Gain=1e+4
  Product : Product
  Product1 : Product
  Subtract : Sum
  Subtract1 : Sum
  im : Outport
  wires:
  Gain1/1 -> Product/2
  Product1/1 -> Subtract1/2
  Constant/1 -> Subtract1/1
  q/1 -> Product/1, Divide/2, Gain1/1
  Divide/1 -> im/1
  Subtract1/1 -> Divide/3
  Gain/1 -> Subtract/1
  h/1 -> Gain/1
  eta/1 -> Gain2/1
  Gain2/1 -> Product1/1
  um/1 -> Product1/2
  Product/1 -> Subtract/2
  Subtract/1 -> Divide/1

== system proiect_date_modificateV2/pert_pompa_pt_feedforward/Filtru  ==
  q : Inport
  Integrator : Integrator  InitialCondition=29.2
  Sum : Sum  Inputs=|+-
  "q_f " : Outport
  wires:
  q/1 -> Sum/1
  Sum/1 -> Integrator/1
  Integrator/1 -> Sum/2, "q_f "/1

== system proiect_date_modificateV2/pert_pompa_pt_feedforward/Motor ==
  um : Inport
  im : Inport  Port=2
  "Add " : Sum  Inputs=+-
  "Rm " : Gain  Gain=3
  kn : Outport
  wires:
  um/1 -> "Add "/1
  "Add "/1 -> kn/1
  "Rm "/1 -> "Add "/2
  im/1 -> "Rm "/1

== system proiect_date_modificateV2/pert_pompa_pt_feedforward/Randament ==
  q : Inport
  um : Inport  Port=2
  Gain : Gain  Gain=keta
  Product : Product
  eta : Outport
  wires:
  Product/1 -> eta/1
  um/1 -> Gain/1
  Gain/1 -> Product/2
  q/1 -> Product/1

== system proiect_date_modificateV2/pert_pompa_pt_feedforward/Rezervor ==
  "q " : Inport
  Fcn : Fcn  Expr=sqrt(u)*9
  Gain : Gain  Gain=1/332.5
  Integrator : Integrator  InitialCondition=10.5
  Sum : Sum  Inputs=|+-
  h : Outport
  wires:
  Gain/1 -> Integrator/1
  "q "/1 -> Sum/1
  Integrator/1 -> h/1, Fcn/1
  Sum/1 -> Gain/1
  Fcn/1 -> Sum/2

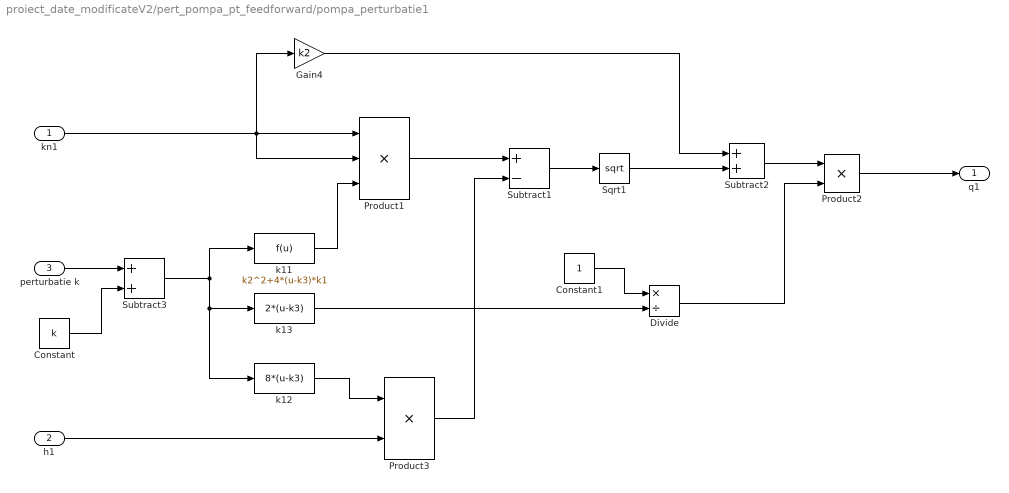
== system proiect_date_modificateV2/pert_pompa_pt_feedforward/pompa_perturbatie1 ==
  kn1 : Inport
  h1 : Inport  Port=2
  perturbatie k : Inport  Port=3
  Constant : Constant  Value=k
  Constant1 : Constant
  Divide : Product  Inputs=*/
  Gain4 : Gain  Gain=k2
  Product1 : Product  Inputs=3
  Product2 : Product
  Product3 : Product
  Sqrt1 : Sqrt
  Subtract1 : Sum  Inputs=+-
  Subtract2 : Sum
  Subtract3 : Sum
  k11 : Fcn  Expr=k2^2+4*(u-k3)*k1
  k12 : Fcn  Expr=8*(u-k3)
  k13 : Fcn  Expr=2*(u-k3)
  q1 : Outport
  wires:
  kn1/1 -> Gain4/1, Product1/1, Product1/2
  Sqrt1/1 -> Subtract2/2
  Product1/1 -> Subtract1/1
  Product3/1 -> Subtract1/2
  Constant1/1 -> Divide/1
  Subtract2/1 -> Product2/1
  k11/1 -> Product1/3
  Divide/1 -> Product2/2
  perturbatie k/1 -> Subtract3/1
  Subtract1/1 -> Sqrt1/1
  k13/1 -> Divide/2
  h1/1 -> Product3/2
  Product2/1 -> q1/1
  Constant/1 -> Subtract3/2
  Subtract3/1 -> k12/1, k13/1, k11/1
  k12/1 -> Product3/1
  Gain4/1 -> Subtract2/1

== system proiect_date_modificateV2/sistem bucla inchisa perturbatie/Amplificator ==
  ua : Inport
  Constant : Constant  Value=8.1
  Gain : Gain  Gain=2.2
  Gain1 : Gain  Gain=5
  Gain2 : Gain  Gain=2.2
  Saturation : Saturate  UpperLimit=22  LowerLimit=0
  Sum : Sum  Inputs=|++
  Sum1 : Sum  Inputs=|+-
  Switch : Switch  Threshold=8.1  SaturateOnIntegerOverflow=off  InputSameDT=off
  um : Outport
  wires:
  Switch/1 -> Saturation/1
  ua/1 -> Switch/2, Gain/1, Gain2/1, Sum1/1
  Sum/1 -> Switch/1
  Gain2/1 -> Sum/1
  Gain/1 -> Switch/3
  Saturation/1 -> um/1
  Gain1/1 -> Sum/2
  Sum1/1 -> Gain1/1
  Constant/1 -> Sum1/2

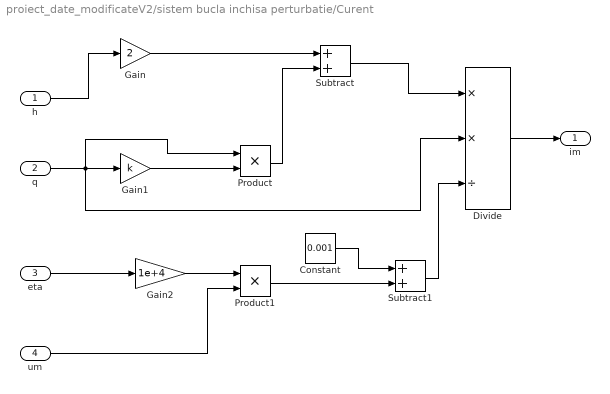
== system proiect_date_modificateV2/sistem bucla inchisa perturbatie/Curent ==
  h : Inport
  q : Inport  Port=2
  eta : Inport  Port=3
  um : Inport  Port=4
  Constant : Constant  Value=0.001
  Divide : Product  Inputs=**/
  Gain : Gain  Gain=2
  Gain1 : Gain  Gain=k
  Gain2 : Gain  Gain=1e+4
  Product : Product
  Product1 : Product
  Subtract : Sum
  Subtract1 : Sum
  im : Outport
  wires:
  Gain1/1 -> Product/2
  Product1/1 -> Subtract1/2
  Constant/1 -> Subtract1/1
  q/1 -> Product/1, Divide/2, Gain1/1
  Divide/1 -> im/1
  Subtract1/1 -> Divide/3
  Gain/1 -> Subtract/1
  h/1 -> Gain/1
  eta/1 -> Gain2/1
  Gain2/1 -> Product1/1
  um/1 -> Product1/2
  Product/1 -> Subtract/2
  Subtract/1 -> Divide/1

== system proiect_date_modificateV2/sistem bucla inchisa perturbatie/Filtru  ==
  q : Inport
  Integrator : Integrator  InitialCondition=29.2
  Sum : Sum  Inputs=|+-
  "q_f " : Outport
  wires:
  q/1 -> Sum/1
  Sum/1 -> Integrator/1
  Integrator/1 -> Sum/2, "q_f "/1

== system proiect_date_modificateV2/sistem bucla inchisa perturbatie/Motor ==
  um : Inport
  im : Inport  Port=2
  "Add " : Sum  Inputs=+-
  "Rm " : Gain  Gain=3
  kn : Outport
  wires:
  um/1 -> "Add "/1
  "Add "/1 -> kn/1
  "Rm "/1 -> "Add "/2
  im/1 -> "Rm "/1

== system proiect_date_modificateV2/sistem bucla inchisa perturbatie/Pompa  ==
  kn : Inport
  h : Inport  Port=2
  Gain : Gain  Gain=k2
  Gain1 : Gain  Gain=k11
  Gain2 : Gain  Gain=k12
  Gain3 : Gain  Gain=1/k13
  Product : Product
  Sqrt : Sqrt
  Subtract1 : Sum  Inputs=+-
  substract : Sum
  q : Outport
  wires:
  Gain3/1 -> q/1
  Subtract1/1 -> Sqrt/1
  Gain/1 -> substract/1
  h/1 -> Gain2/1
  Product/1 -> Gain1/1
  Gain1/1 -> Subtract1/1
  Gain2/1 -> Subtract1/2
  Sqrt/1 -> substract/2
  kn/1 -> Gain/1, Product/2, Product/1
  substract/1 -> Gain3/1

== system proiect_date_modificateV2/sistem bucla inchisa perturbatie/Randament ==
  q : Inport
  um : Inport  Port=2
  Gain : Gain  Gain=keta
  Product : Product
  eta : Outport
  wires:
  Product/1 -> eta/1
  um/1 -> Gain/1
  Gain/1 -> Product/2
  q/1 -> Product/1

== system proiect_date_modificateV2/sistem bucla inchisa perturbatie/Rezervor cu perturbatie ==
  q1 : Inport
  C : Step  Time=250  Before=C  After=11  SampleTime=0
  Gain : Gain  Gain=1/332.5
  Integrator : Integrator  InitialCondition=10.5
  Product : Product
  Sqrt : Sqrt
  Sum : Sum  Inputs=|+-
  h1 : Outport
  wires:
  Integrator/1 -> h1/1, Sqrt/1
  q1/1 -> Sum/1
  Sum/1 -> Gain/1
  Gain/1 -> Integrator/1
  Product/1 -> Sum/2
  C/1 -> Product/2
  Sqrt/1 -> Product/1

== system proiect_date_modificateV2/sistem1/Amplificator ==
  ua : Inport
  Constant : Constant  Value=8.1
  Gain : Gain  Gain=2.2
  Gain1 : Gain  Gain=2.2
  Gain2 : Gain  Gain=5
  Saturation : Saturate  UpperLimit=22  LowerLimit=0
  Sum : Sum  Inputs=|+-
  Sum1 : Sum  Inputs=|++
  Switch : Switch  Threshold=8.1  SaturateOnIntegerOverflow=off  InputSameDT=off
  um : Outport
  wires:
  ua/1 -> Sum/1, Gain1/1, Switch/2, Gain/1
  Sum1/1 -> Switch/1
  Gain/1 -> Switch/3
  Sum/1 -> Gain2/1
  Constant/1 -> Sum/2
  Switch/1 -> Saturation/1
  Gain1/1 -> Sum1/1
  Gain2/1 -> Sum1/2
  Saturation/1 -> um/1

== system proiect_date_modificateV2/sistem1/Bazin ==
  q : Inport
  Fcn : Fcn  Expr=sqrt(u)*7.55
  Gain : Gain  Gain=1/332.5
  Integrator : Integrator
  Sum : Sum  Inputs=|+-
  h : Outport
  wires:
  Integrator/1 -> h/1, Fcn/1
  Fcn/1 -> Sum/2
  Gain/1 -> Integrator/1
  q/1 -> Sum/1
  Sum/1 -> Gain/1

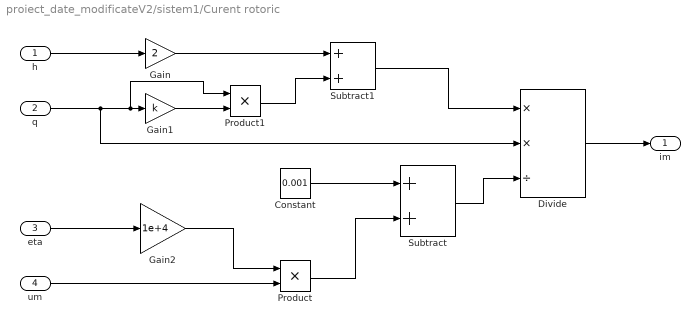
== system proiect_date_modificateV2/sistem1/Curent rotoric ==
  h : Inport
  q : Inport  Port=2
  eta : Inport  Port=3
  um : Inport  Port=4
  Constant : Constant  Value=0.001
  Divide : Product  Inputs=**/
  Gain : Gain  Gain=2
  Gain1 : Gain  Gain=k
  Gain2 : Gain  Gain=1e+4
  Product : Product
  Product1 : Product
  Subtract : Sum
  Subtract1 : Sum
  im : Outport
  wires:
  Subtract/1 -> Divide/3
  Divide/1 -> im/1
  h/1 -> Gain/1
  um/1 -> Product/2
  q/1 -> Divide/2, Product1/1, Gain1/1
  Constant/1 -> Subtract/1
  Product/1 -> Subtract/2
  eta/1 -> Gain2/1
  Gain2/1 -> Product/1
  Gain/1 -> Subtract1/1
  Subtract1/1 -> Divide/1
  Gain1/1 -> Product1/2
  Product1/1 -> Subtract1/2

== system proiect_date_modificateV2/sistem1/Filtru ==
  q : Inport
  Integrator : Integrator
  Sum : Sum  Inputs=|+-
  qf : Outport
  wires:
  Integrator/1 -> qf/1, Sum/2
  q/1 -> Sum/1
  Sum/1 -> Integrator/1

== system proiect_date_modificateV2/sistem1/Motor ==
  um : Inport
  im : Inport  Port=2
  Add : Sum  Inputs=+-
  Rm : Gain  Gain=3
  kn : Outport
  wires:
  Rm/1 -> Add/2
  um/1 -> Add/1
  im/1 -> Rm/1
  Add/1 -> kn/1

== system proiect_date_modificateV2/sistem1/Pompa ==
  kn : Inport
  h : Inport  Port=2
  Gain : Gain  Gain=k2
  Gain1 : Gain  Gain=1/k13
  Gain2 : Gain  Gain=k11
  Gain3 : Gain  Gain=k12
  Product : Product
  Sqrt : Sqrt
  Subtract : Sum  Inputs=+-
  Subtract1 : Sum
  q : Outport
  wires:
  kn/1 -> Gain/1, Product/1, Product/2
  Gain/1 -> Subtract1/1
  Product/1 -> Gain2/1
  Subtract/1 -> Sqrt/1
  Gain3/1 -> Subtract/2
  Gain2/1 -> Subtract/1
  h/1 -> Gain3/1
  Sqrt/1 -> Subtract1/2
  Subtract1/1 -> Gain1/1
  Gain1/1 -> q/1

== system proiect_date_modificateV2/sistem1/Randament pompa ==
  q : Inport
  um : Inport  Port=2
  Gain : Gain  Gain=keta
  Product : Product
  eta : Outport
  wires:
  Gain/1 -> Product/2
  um/1 -> Gain/1
  Product/1 -> eta/1
  q/1 -> Product/1

== system proiect_date_modificateV2/Cascada/sistem_cascada/Amplificator  ==
  ua : Inport
  Constant : Constant  Value=8.1
  Gain : Gain  Gain=2.2
  Gain1 : Gain  Gain=5
  Gain2 : Gain  Gain=2.2
  Saturation : Saturate  UpperLimit=22  LowerLimit=0
  Sum : Sum  Inputs=|+-
  Sum1 : Sum  Inputs=|++
  Switch : Switch  Threshold=8.1  SaturateOnIntegerOverflow=off  InputSameDT=off
  um : Outport
  wires:
  Gain/1 -> Switch/3
  Gain1/1 -> Sum1/2
  Switch/1 -> Saturation/1
  Constant/1 -> Sum/2
  Gain2/1 -> Sum1/1
  Sum/1 -> Gain1/1
  Saturation/1 -> um/1
  ua/1 -> Sum/1, Gain2/1, Gain/1, Switch/2
  Sum1/1 -> Switch/1

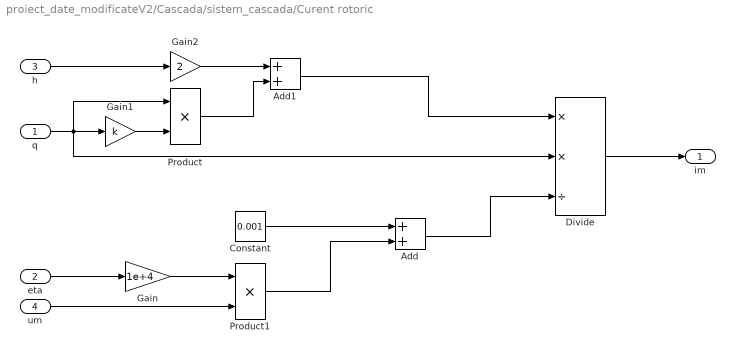
== system proiect_date_modificateV2/Cascada/sistem_cascada/Curent rotoric ==
  q : Inport
  eta : Inport  Port=2
  h : Inport  Port=3
  um : Inport  Port=4
  Add : Sum
  Add1 : Sum
  Constant : Constant  Value=0.001
  Divide : Product  Inputs=**/
  Gain : Gain  Gain=1e+4
  Gain1 : Gain  Gain=k
  Gain2 : Gain  Gain=2
  Product : Product
  Product1 : Product
  im : Outport
  wires:
  Add1/1 -> Divide/1
  Constant/1 -> Add/1
  Add/1 -> Divide/3
  Gain1/1 -> Product/2
  Product/1 -> Add1/2
  um/1 -> Product1/2
  Product1/1 -> Add/2
  Divide/1 -> im/1
  Gain/1 -> Product1/1
  Gain2/1 -> Add1/1
  eta/1 -> Gain/1
  q/1 -> Divide/2, Product/1, Gain1/1
  h/1 -> Gain2/1

== system proiect_date_modificateV2/Cascada/sistem_cascada/Filtru ==
  q : Inport
  Integrator : Integrator  InitialCondition=29.2
  Sum : Sum  Inputs=|+-
  h : Outport
  wires:
  Sum/1 -> Integrator/1
  q/1 -> Sum/1
  Integrator/1 -> h/1, Sum/2

== system proiect_date_modificateV2/Cascada/sistem_cascada/Motor ==
  um : Inport
  im : Inport  Port=2
  Add : Sum  Inputs=+-
  "Rm " : Gain  Gain=3
  kn : Outport
  wires:
  "Rm "/1 -> Add/2
  Add/1 -> kn/1
  um/1 -> Add/1
  im/1 -> "Rm "/1

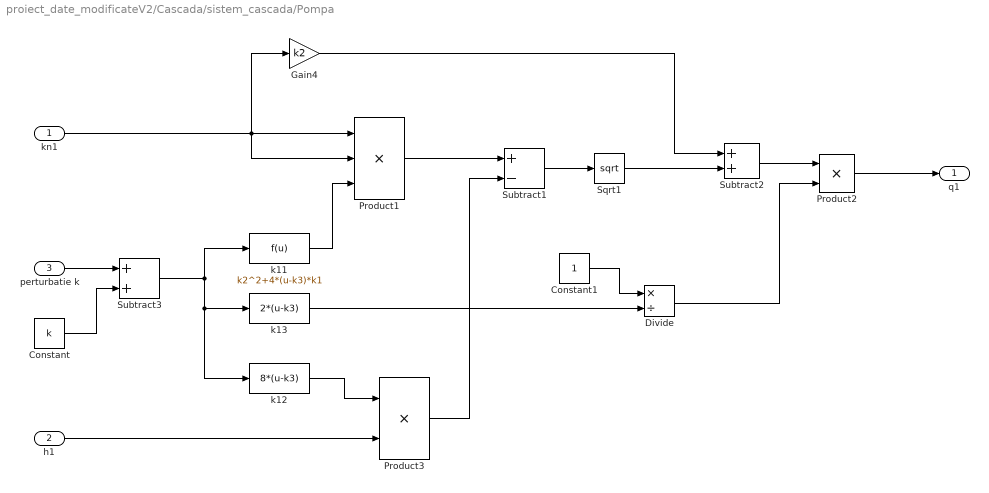
== system proiect_date_modificateV2/Cascada/sistem_cascada/Pompa ==
  kn1 : Inport
  h1 : Inport  Port=2
  perturbatie k : Inport  Port=3
  Constant : Constant  Value=k
  Constant1 : Constant
  Divide : Product  Inputs=*/
  Gain4 : Gain  Gain=k2
  Product1 : Product  Inputs=3
  Product2 : Product
  Product3 : Product
  Sqrt1 : Sqrt
  Subtract1 : Sum  Inputs=+-
  Subtract2 : Sum
  Subtract3 : Sum
  k11 : Fcn  Expr=k2^2+4*(u-k3)*k1
  k12 : Fcn  Expr=8*(u-k3)
  k13 : Fcn  Expr=2*(u-k3)
  q1 : Outport
  wires:
  kn1/1 -> Gain4/1, Product1/1, Product1/2
  Subtract1/1 -> Sqrt1/1
  Gain4/1 -> Subtract2/1
  Sqrt1/1 -> Subtract2/2
  perturbatie k/1 -> Subtract3/1
  Constant/1 -> Subtract3/2
  Product2/1 -> q1/1
  Subtract2/1 -> Product2/1
  Divide/1 -> Product2/2
  Constant1/1 -> Divide/1
  Product1/1 -> Subtract1/1
  h1/1 -> Product3/2
  Product3/1 -> Subtract1/2
  k11/1 -> Product1/3
  Subtract3/1 -> k12/1, k13/1, k11/1
  k12/1 -> Product3/1
  k13/1 -> Divide/2

== system proiect_date_modificateV2/Cascada/sistem_cascada/Randament ==
  q : Inport
  um : Inport  Port=2
  Gain : Gain  Gain=keta
  Product : Product
  eta : Outport
  wires:
  Gain/1 -> Product/2
  Product/1 -> eta/1
  q/1 -> Product/1
  um/1 -> Gain/1

== system proiect_date_modificateV2/Cascada/sistem_cascada/Rezervor ==
  q : Inport
  Fcn : Fcn  Expr=sqrt(u)*9
  Gain : Gain  Gain=1/332.5
  Integrator : Integrator  InitialCondition=10.5
  Sum : Sum  Inputs=|+-
  h : Outport
  wires:
  q/1 -> Sum/1
  Sum/1 -> Gain/1
  Integrator/1 -> h/1, Fcn/1
  Fcn/1 -> Sum/2
  Gain/1 -> Integrator/1

== system proiect_date_modificateV2/Cascada+FF/cascada+ff/Amplificator  ==
  ua : Inport
  Constant : Constant  Value=8.1
  Gain : Gain  Gain=2.2
  Gain1 : Gain  Gain=5
  Gain2 : Gain  Gain=2.2
  Saturation : Saturate  UpperLimit=22  LowerLimit=0
  Sum : Sum  Inputs=|+-
  Sum1 : Sum  Inputs=|++
  Switch : Switch  Threshold=8.1  SaturateOnIntegerOverflow=off  InputSameDT=off
  um : Outport
  wires:
  Gain/1 -> Switch/3
  Gain1/1 -> Sum1/2
  Switch/1 -> Saturation/1
  Constant/1 -> Sum/2
  Gain2/1 -> Sum1/1
  Sum/1 -> Gain1/1
  Saturation/1 -> um/1
  ua/1 -> Sum/1, Gain2/1, Gain/1, Switch/2
  Sum1/1 -> Switch/1

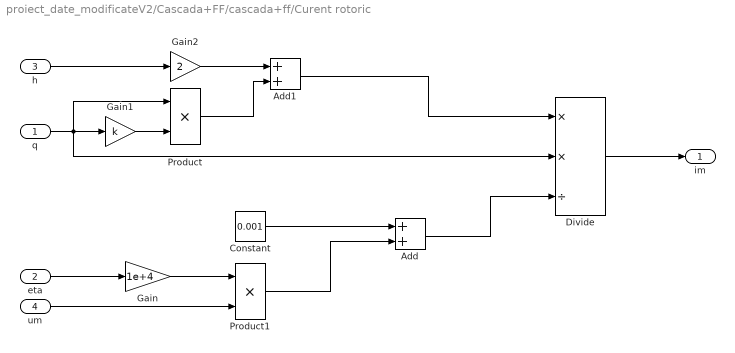
== system proiect_date_modificateV2/Cascada+FF/cascada+ff/Curent rotoric ==
  q : Inport
  eta : Inport  Port=2
  h : Inport  Port=3
  um : Inport  Port=4
  Add : Sum
  Add1 : Sum
  Constant : Constant  Value=0.001
  Divide : Product  Inputs=**/
  Gain : Gain  Gain=1e+4
  Gain1 : Gain  Gain=k
  Gain2 : Gain  Gain=2
  Product : Product
  Product1 : Product
  im : Outport
  wires:
  Add1/1 -> Divide/1
  Constant/1 -> Add/1
  Add/1 -> Divide/3
  Gain1/1 -> Product/2
  Product/1 -> Add1/2
  um/1 -> Product1/2
  Product1/1 -> Add/2
  Divide/1 -> im/1
  Gain/1 -> Product1/1
  Gain2/1 -> Add1/1
  eta/1 -> Gain/1
  q/1 -> Divide/2, Product/1, Gain1/1
  h/1 -> Gain2/1

== system proiect_date_modificateV2/Cascada+FF/cascada+ff/Filtru ==
  q : Inport
  Integrator : Integrator  InitialCondition=29.2
  Sum : Sum  Inputs=|+-
  h : Outport
  wires:
  Sum/1 -> Integrator/1
  q/1 -> Sum/1
  Integrator/1 -> h/1, Sum/2

== system proiect_date_modificateV2/Cascada+FF/cascada+ff/Motor ==
  um : Inport
  im : Inport  Port=2
  Add : Sum  Inputs=+-
  "Rm " : Gain  Gain=3
  kn : Outport
  wires:
  "Rm "/1 -> Add/2
  Add/1 -> kn/1
  um/1 -> Add/1
  im/1 -> "Rm "/1

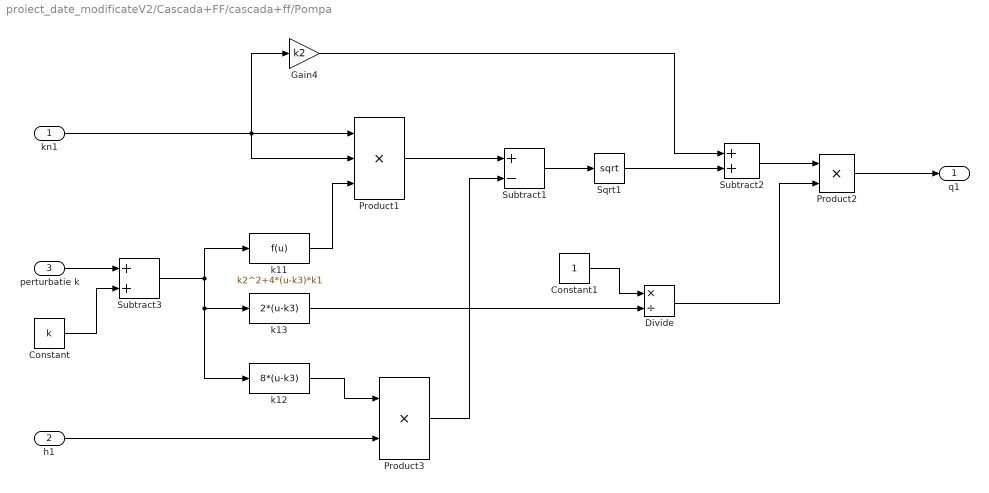
== system proiect_date_modificateV2/Cascada+FF/cascada+ff/Pompa ==
  kn1 : Inport
  h1 : Inport  Port=2
  perturbatie k : Inport  Port=3
  Constant : Constant  Value=k
  Constant1 : Constant
  Divide : Product  Inputs=*/
  Gain4 : Gain  Gain=k2
  Product1 : Product  Inputs=3
  Product2 : Product
  Product3 : Product
  Sqrt1 : Sqrt
  Subtract1 : Sum  Inputs=+-
  Subtract2 : Sum
  Subtract3 : Sum
  k11 : Fcn  Expr=k2^2+4*(u-k3)*k1
  k12 : Fcn  Expr=8*(u-k3)
  k13 : Fcn  Expr=2*(u-k3)
  q1 : Outport
  wires:
  kn1/1 -> Gain4/1, Product1/1, Product1/2
  Subtract1/1 -> Sqrt1/1
  Gain4/1 -> Subtract2/1
  Sqrt1/1 -> Subtract2/2
  perturbatie k/1 -> Subtract3/1
  Constant/1 -> Subtract3/2
  Product2/1 -> q1/1
  Subtract2/1 -> Product2/1
  Divide/1 -> Product2/2
  Constant1/1 -> Divide/1
  Product1/1 -> Subtract1/1
  h1/1 -> Product3/2
  Product3/1 -> Subtract1/2
  k11/1 -> Product1/3
  Subtract3/1 -> k12/1, k13/1, k11/1
  k12/1 -> Product3/1
  k13/1 -> Divide/2

== system proiect_date_modificateV2/Cascada+FF/cascada+ff/Randament ==
  q : Inport
  um : Inport  Port=2
  Gain : Gain  Gain=keta
  Product : Product
  eta : Outport
  wires:
  Gain/1 -> Product/2
  Product/1 -> eta/1
  q/1 -> Product/1
  um/1 -> Gain/1

== system proiect_date_modificateV2/Cascada+FF/cascada+ff/Rezervor ==
  q : Inport
  Fcn : Fcn  Expr=sqrt(u)*9
  Gain : Gain  Gain=1/332.5
  Integrator : Integrator  InitialCondition=10.5
  Sum : Sum  Inputs=|+-
  h : Outport
  wires:
  q/1 -> Sum/1
  Sum/1 -> Gain/1
  Integrator/1 -> h/1, Fcn/1
  Fcn/1 -> Sum/2
  Gain/1 -> Integrator/1

== system proiect_date_modificateV2/FF/sistem_feedforward/Amplificator ==
  ua : Inport
  Constant : Constant  Value=8.1
  Gain : Gain  Gain=2.2
  Gain1 : Gain  Gain=5
  Gain2 : Gain  Gain=2.2
  Saturation : Saturate  UpperLimit=22  LowerLimit=0
  Sum : Sum  Inputs=|++
  Sum1 : Sum  Inputs=|+-
  Switch : Switch  Threshold=8.1  SaturateOnIntegerOverflow=off  InputSameDT=off
  um : Outport
  wires:
  Switch/1 -> Saturation/1
  ua/1 -> Switch/2, Gain/1, Gain2/1, Sum1/1
  Sum/1 -> Switch/1
  Gain2/1 -> Sum/1
  Gain/1 -> Switch/3
  Saturation/1 -> um/1
  Gain1/1 -> Sum/2
  Sum1/1 -> Gain1/1
  Constant/1 -> Sum1/2

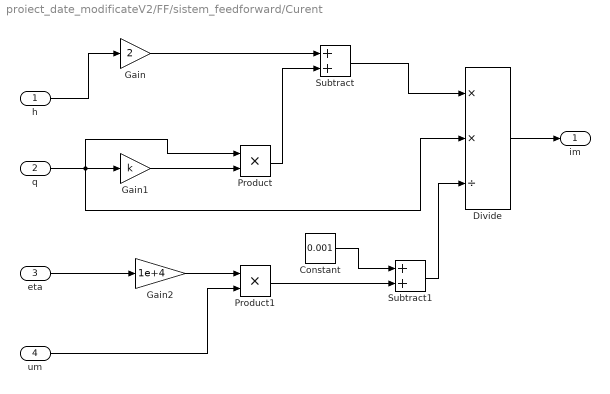
== system proiect_date_modificateV2/FF/sistem_feedforward/Curent ==
  h : Inport
  q : Inport  Port=2
  eta : Inport  Port=3
  um : Inport  Port=4
  Constant : Constant  Value=0.001
  Divide : Product  Inputs=**/
  Gain : Gain  Gain=2
  Gain1 : Gain  Gain=k
  Gain2 : Gain  Gain=1e+4
  Product : Product
  Product1 : Product
  Subtract : Sum
  Subtract1 : Sum
  im : Outport
  wires:
  Gain1/1 -> Product/2
  Product1/1 -> Subtract1/2
  Constant/1 -> Subtract1/1
  q/1 -> Product/1, Divide/2, Gain1/1
  Divide/1 -> im/1
  Subtract1/1 -> Divide/3
  Gain/1 -> Subtract/1
  h/1 -> Gain/1
  eta/1 -> Gain2/1
  Gain2/1 -> Product1/1
  um/1 -> Product1/2
  Product/1 -> Subtract/2
  Subtract/1 -> Divide/1

== system proiect_date_modificateV2/FF/sistem_feedforward/Filtru  ==
  q : Inport
  Integrator : Integrator  InitialCondition=29.2
  Sum : Sum  Inputs=|+-
  "q_f " : Outport
  wires:
  q/1 -> Sum/1
  Sum/1 -> Integrator/1
  Integrator/1 -> Sum/2, "q_f "/1

== system proiect_date_modificateV2/FF/sistem_feedforward/Motor ==
  um : Inport
  im : Inport  Port=2
  "Add " : Sum  Inputs=+-
  "Rm " : Gain  Gain=3
  kn : Outport
  wires:
  um/1 -> "Add "/1
  "Add "/1 -> kn/1
  "Rm "/1 -> "Add "/2
  im/1 -> "Rm "/1
